simulink model "scheme3"  (R2024a)
settings: Solver=VariableStepAuto  StartTime=0.0  StopTime=10.0  RelTol=1e-8
undefined symbols (not defined in the file or in its folder): A, Abebra, B, Bf, C, Cz, D, Dz, e0, Gamma, K1, K2, L, wfen, x0
settings Model: Creator=alexivanov  LastModifiedBy=alexivanov

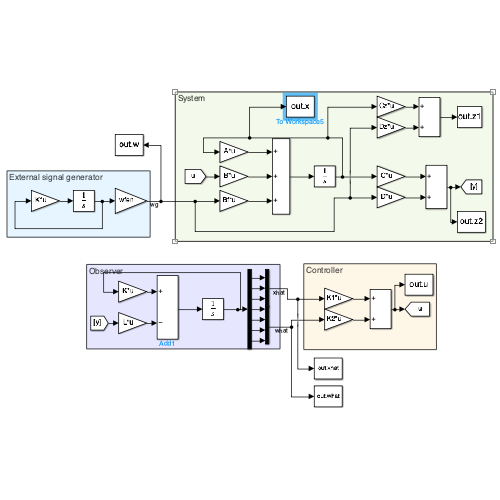
[thumbnail: Simulink's stored preview of the top-level diagram]
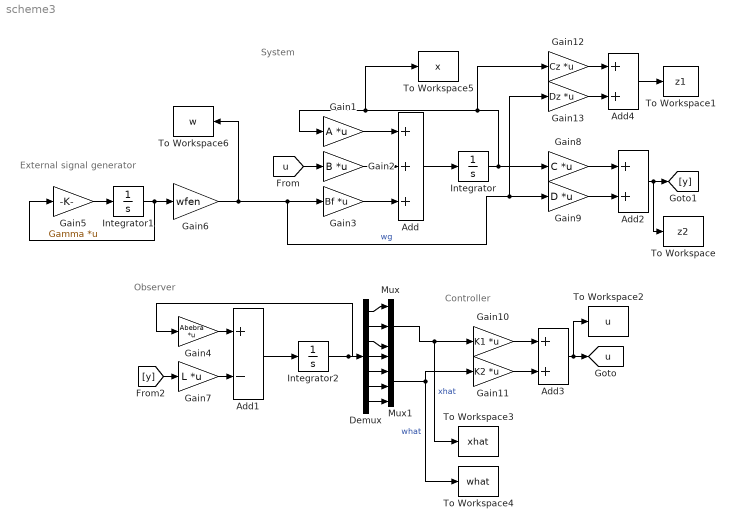
== system scheme3 ==
  note: System
  note: Controller
  note: Observer
  note: External signal generator
  Add : Sum  Inputs=+++
  Add1 : Sum  Inputs=+-
  Add2 : Sum
  Add3 : Sum
  Add4 : Sum
  Demux : Demux  Outputs=7
  Gain1 : Gain  Gain=A  Multiplication=Matrix(K*u)
  Gain10 : Gain  Gain=K1  Multiplication=Matrix(K*u)
  Gain11 : Gain  Gain=K2  Multiplication=Matrix(K*u)
  Gain12 : Gain  Gain=Cz  Multiplication=Matrix(K*u)
  Gain13 : Gain  Gain=Dz  Multiplication=Matrix(K*u)
  Gain2 : Gain  Gain=B  Multiplication=Matrix(K*u)
  Gain3 : Gain  Gain=Bf  Multiplication=Matrix(K*u)
  Gain4 : Gain  Gain=Abebra  Multiplication=Matrix(K*u)
  Gain5 : Gain  Gain=Gamma  Multiplication=Matrix(K*u)
  Gain6 : Gain  Gain=wfen
  Gain7 : Gain  Gain=L  Multiplication=Matrix(K*u)
  Gain8 : Gain  Gain=C  Multiplication=Matrix(K*u)
  Gain9 : Gain  Gain=D  Multiplication=Matrix(K*u)
  Integrator : Integrator  InitialCondition=x0
  Integrator1 : Integrator  InitialCondition=[1; 1; 1; 1]
  Integrator2 : Integrator  InitialCondition=e0
  Mux : Mux  Inputs=3
  Mux1 : Mux
  To Workspace : ToWorkspace  VariableName=z2  SampleTime=-1
  To Workspace1 : ToWorkspace  VariableName=z1  SampleTime=-1
  To Workspace2 : ToWorkspace  VariableName=u  SampleTime=-1
  To Workspace3 : ToWorkspace  VariableName=xhat  SampleTime=-1
  To Workspace4 : ToWorkspace  VariableName=what  SampleTime=-1
  To Workspace5 : ToWorkspace  VariableName=x  SampleTime=-1
  To Workspace6 : ToWorkspace  VariableName=w  SampleTime=-1
  tag scope: u=global
  wires:
  Integrator1/1 -> Gain5/1, Gain6/1
  Gain5/1 -> Integrator1/1
  Gain2/1 -> Add/2
  Gain3/1 -> Add/3
  Gain1/1 -> Add/1
  Gain6/1 -> To Workspace6/1, Gain13/1, Gain9/1, Gain3/1  "wg"
  Add/1 -> Integrator/1
  Integrator/1 -> Gain8/1, Gain12/1, To Workspace5/1, Gain1/1
  Integrator2/1 -> Gain4/1, Demux/1
  Gain4/1 -> Add1/1
  Gain7/1 -> Add1/2
  Add1/1 -> Integrator2/1
  Gain8/1 -> Add2/1
  Gain9/1 -> Add2/2
  [u] -> Gain2/1
  [y] -> Gain7/1
  Add2/1 -> To Workspace/1, [y]
  Gain10/1 -> Add3/1
  Gain11/1 -> Add3/2
  Add3/1 -> To Workspace2/1, [u]
  Add4/1 -> To Workspace1/1
  Gain12/1 -> Add4/1
  Gain13/1 -> Add4/2
  Demux/2 -> Mux/2
  Demux/1 -> Mux/1
  Demux/3 -> Mux/3
  Demux/4 -> Mux1/1
  Demux/5 -> Mux1/2
  Demux/6 -> Mux1/3
  Demux/7 -> Mux1/4
  Mux1/1 -> To Workspace4/1, Gain11/1  "what"
  Mux/1 -> Gain10/1, To Workspace3/1  "xhat"
